simulink model "Lab_4_EBD_ibrahim"  (R2016b)
settings: Solver=VariableStepAuto  StartTime=0.0  StopTime=6  MaxStep=0.00005  RelTol=1e-3
undefined symbols (not defined in the file): F_human_max, F_rated_wheel, k, Lever_ratio, P_servo_max, R_master, R_servo, s_rated_wheel, V_initial
libraries: sdl_lib x9, nesl_utility x6, simulink x1
settings Model: Creator=AHMED MOHSEN  LastModifiedBy=AHMED MOHSEN
settings DataIOCC: ReturnWorkspaceOutputs=on
settings DebuggingCC: UnconnectedInputMsg=none  UnconnectedOutputMsg=none  UnconnectedLineMsg=none
settings ModelReferenceCC: EnableRefExpFcnMdlSchedulingChecks=off
settings SFSimCC: SimUseLocalCustomCode=on
settings RTWCC: RTWUseLocalCustomCode=on

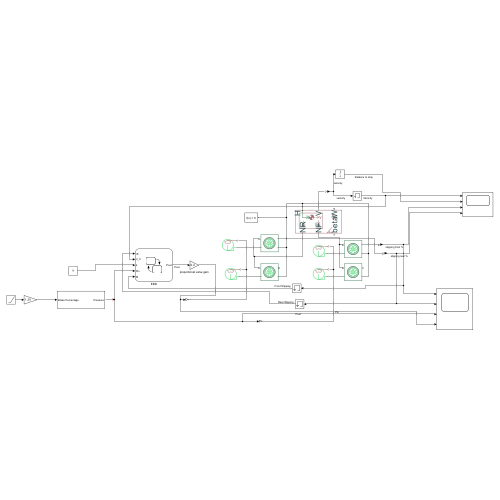
[thumbnail: Simulink's stored preview of the top-level diagram]
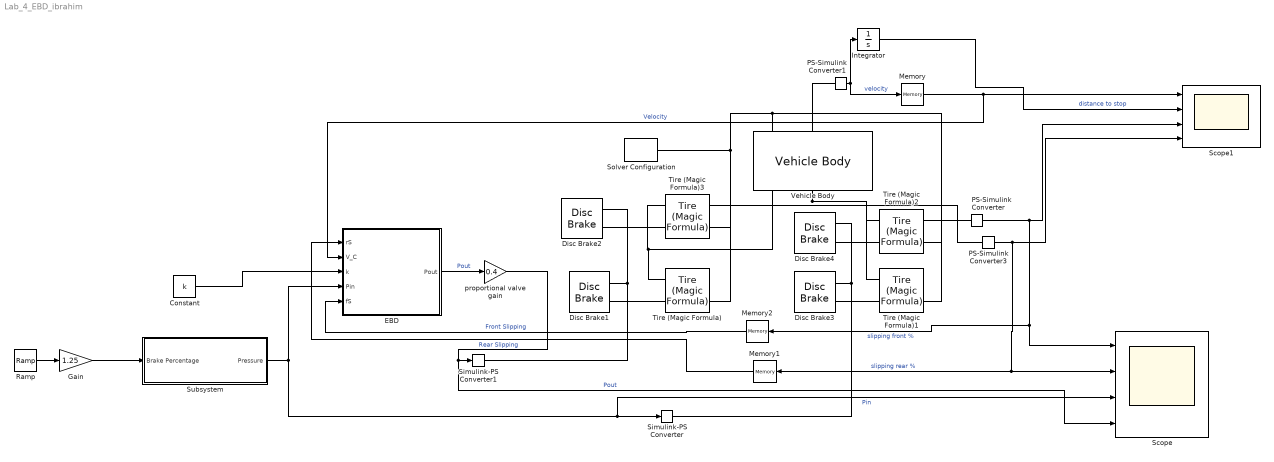
== system Lab_4_EBD_ibrahim ==
  Constant : Constant  Value=k
  Disc Brake1 : sdl_lib/Brakes & Detents/Rotational/Disc Brake  r_mean=R_disk mm  bore=D_cylinder mm  n_pads=2  thermal_port=simscape.enum.thermaleffects.omit  mu_static=0.9  mu_coulomb=0.7  temperature_TLU=[280, 300, 320] K  mu_static_TLU=[.9, .8, .7]  mu_coulomb_TLU=[.8, .7, .6]  brkwy_vel=0.1 rad/s  visc_coef=Visc_coeff N*m*s/rad  enable_faults=simscape.enum.onoff.off  faulted_pressure=0 bar  external_fault=simscape.enum.onoff.off  temporal_fault=simscape.enum.onoff.off  fault_time=5 s  report_fault=simscape.enum.assert.action.none  thermal_mass=50 kJ/K  temperature_specify=off  temperature_priority=High  temperature=300 K  temperature_nominal_specify=off  temperature_nominal_unit=K  temperature_nominal_value=1
  Disc Brake2 : sdl_lib/Brakes & Detents/Rotational/Disc Brake  r_mean=R_disk mm  bore=D_cylinder mm  n_pads=2  thermal_port=simscape.enum.thermaleffects.omit  mu_static=0.9  mu_coulomb=0.7  temperature_TLU=[280, 300, 320] K  mu_static_TLU=[.9, .8, .7]  mu_coulomb_TLU=[.8, .7, .6]  brkwy_vel=0.1 rad/s  visc_coef=Visc_coeff N*m*s/rad  enable_faults=simscape.enum.onoff.off  faulted_pressure=0 bar  external_fault=simscape.enum.onoff.off  temporal_fault=simscape.enum.onoff.off  fault_time=5 s  report_fault=simscape.enum.assert.action.none  thermal_mass=50 kJ/K  temperature_specify=off  temperature_priority=High  temperature=300 K  temperature_nominal_specify=off  temperature_nominal_unit=K  temperature_nominal_value=1
  Disc Brake3 : sdl_lib/Brakes & Detents/Rotational/Disc Brake  r_mean=R_disk mm  bore=D_cylinder mm  n_pads=2  thermal_port=simscape.enum.thermaleffects.omit  mu_static=0.9  mu_coulomb=0.7  temperature_TLU=[280, 300, 320] K  mu_static_TLU=[.9, .8, .7]  mu_coulomb_TLU=[.8, .7, .6]  brkwy_vel=0.1 rad/s  visc_coef=Visc_coeff N*m*s/rad  enable_faults=simscape.enum.onoff.off  faulted_pressure=0 bar  external_fault=simscape.enum.onoff.off  temporal_fault=simscape.enum.onoff.off  fault_time=5 s  report_fault=simscape.enum.assert.action.none  thermal_mass=50 kJ/K  temperature_specify=off  temperature_priority=High  temperature=300 K  temperature_nominal_specify=off  temperature_nominal_unit=K  temperature_nominal_value=1
  Disc Brake4 : sdl_lib/Brakes & Detents/Rotational/Disc Brake  r_mean=R_disk mm  bore=D_cylinder mm  n_pads=NO_brake_pads  thermal_port=simscape.enum.thermaleffects.omit  mu_static=0.9  mu_coulomb=0.7  temperature_TLU=[280, 300, 320] K  mu_static_TLU=[.9, .8, .7]  mu_coulomb_TLU=[.8, .7, .6]  brkwy_vel=0.1 rad/s  visc_coef=Visc_coeff N*m*s/rad  enable_faults=simscape.enum.onoff.off  faulted_pressure=0 bar  external_fault=simscape.enum.onoff.off  temporal_fault=simscape.enum.onoff.off  fault_time=5 s  report_fault=simscape.enum.assert.action.none  thermal_mass=50 kJ/K  temperature_specify=off  temperature_priority=High  temperature=300 K  temperature_nominal_specify=off  temperature_nominal_unit=K  temperature_nominal_value=1
  EBD : Stateflow chart  TreatAsAtomicUnit=on
  Gain : Gain  Gain=1.25
  Integrator : Integrator
  Memory : Memory  X0=V_initial/3.6  InheritSampleTime=on
  Memory1 : Memory  InheritSampleTime=on
  Memory2 : Memory  InheritSampleTime=on
  PS-Simulink Converter : nesl_utility/PS-Simulink Converter  PhysicalDomain=network_engine_domain  SubClassName=ps_output  LeftPortType=input  RightPortType=output  PseudoPeriodic=off  Frequencies=[]  VectorFormat=1-D array  Unit=inherit  AffineConversion=off
  PS-Simulink Converter1 : nesl_utility/PS-Simulink Converter  PhysicalDomain=network_engine_domain  SubClassName=ps_output  LeftPortType=input  RightPortType=output  PseudoPeriodic=off  Frequencies=[]  VectorFormat=inherit  Unit=m/s  AffineConversion=off
  PS-Simulink Converter3 : nesl_utility/PS-Simulink Converter  PhysicalDomain=network_engine_domain  SubClassName=ps_output  LeftPortType=input  RightPortType=output  PseudoPeriodic=off  Frequencies=[]  VectorFormat=1-D array  Unit=inherit  AffineConversion=off
  Ramp : simulink/Sources/Ramp  slope=1  start=0  X0=0
  Scope : Scope  NumInputPorts=4
  Scope1 : Scope  NumInputPorts=4
  Simulink-PS Converter : nesl_utility/Simulink-PS Converter  PhysicalDomain=network_engine_domain  SubClassName=ps_input  LeftPortType=input  RightPortType=output  PseudoPeriodic=off  Frequencies=[]  NoiseDistribution=none  NoiseParameters=[]  Unit=Pa  AffineConversion=off  FilteringAndDerivatives=provide  SimscapeFilterOrder=1  InputFilterTimeConstant=0.001  UdotUserProvided=0
  Simulink-PS Converter1 : nesl_utility/Simulink-PS Converter  PhysicalDomain=network_engine_domain  SubClassName=ps_input  LeftPortType=input  RightPortType=output  PseudoPeriodic=off  Frequencies=[]  NoiseDistribution=none  NoiseParameters=[]  Unit=Pa  AffineConversion=off  FilteringAndDerivatives=provide  SimscapeFilterOrder=1  InputFilterTimeConstant=0.001  UdotUserProvided=0
  Solver Configuration : nesl_utility/Solver Configuration  PhysicalDomain=network_engine_domain  SubClassName=solver  LeftPortType=input  RightPortType=generic  Tones=[]  Harmonics=[]  SimulateNoise=off  Profile=off  UseLocalSampling=off  EnableSwitchedLinearOptims=on  FrequencyDomain=off  UseCCode=off  RelTol=0.001  AbsTol=0.001  MinStep=1e-09  ToWorkspace=off  RevertToSquareIcSolve=off  NumHomotopyIterations=100  PhasorMode=off  PhasorModeNumHarmonics=1  ConsistencySolver=NEWTON_XTOL_AFTER_FTOL  IndexReductionMethod=DerivativeReplacement  DoDC=off  ResidualTolerance=1e-09  ConsistencyTolSource=GLOBAL  ConsistencyAbsTol=0.001  ConsistencyRelTol=0.001  ConsistencyTolFactor=0.001  UseLocalSolver=off  LocalSolverChoice=NE_BACKWARD_EULER_ADVANCER  ResolveIndetEquations=on  FunctionEvalNumThread=1  LocalSolverSampleTime=0.001  DoFixedCost=off  MaxNonlinIter=3  MaxModeIter=2  ComputeImpulses=off  ImpulseIterations=2  LinearAlgebra=auto  LinearAlgebraNumThread=0  EquationFormulation=NE_TIME_EF  DelaysMemoryBudget=1024  AutomaticFiltering=on  FilteringTimeConstant=0.001  PartitionStorageMethod=AS_NEEDED  PartitionMemoryBudget=1024  PartitionMethod=ROBUST  MultibodyUseLocalSolver=off  MultibodyLocalSolverChoice=ODE1  MultibodyLocalSolverSampleTime=0.001
  Subsystem : Subsystem
  Tire (Magic Formula){,1..3} (4 alike) : sdl_lib/Tires & Vehicles/Tire (Magic Formula)  parameterization=sdl.enum.magic_tire_model.peak  F_z1=F_rated_wheel N  F_x1=F_rated_wheel*s_rated_wheel N  kappa1=10  B_m=10  C_m=1.9  D_m=1  E_m=0.97  fz0=4000 N  p_Cx=1.685  p_Dx=[1.21, -.037]  p_Ex=[.344, .095, -.02, 0]  p_Kx=[21.51, -.163, .245]  p_Hx=[-.002, .002]  p_Vx=[0, 0]  rolling_radius_model=sdl.enum.RollingRadiusParameterization.Constant  r_e=R_wheel m  r_0=0.3 m  breff=8.39  dreff=0.26  freff=0.074  q_re0=0.99  q_v1=0.008  longvl=17 m/s  cz=5e5 N/m  model_resistance=false  resistance_model=sdl.enum.rollingResistanceParameterization.constant  coeff=0.015  p_tire=250e3 Pa  alpha=-0.003  beta=0.97  coeff_a=84e-4  coeff_b=6.2e-4 s/m  coeff_c=1.6e-4 s^2/m^2  p_tire0=240e3 Pa  fz0_resistance=4000 N  vH0=16 m/s  q_Sy=[.0082, 0, .0014, .001, 0, 0, 1.08, -.5]  v_thr=0.001 m/s  enable_scaling_coefficients=false  lfzO=1  lcx=1  lmux=1  lex=1  lkx=1  lhx=1  lvx=1  lmy=1  model_compliance=sdl.enum.compliance.off  stiffness=1e6 N/m  damping=1000 N*s/m  model_inertia=sdl.enum.model_inertia.on  inertia=1 kg*m^2  initial_velocity=V_initial/3.6/R_wheel rad/s  vxlow=1 m/s  v_tr_thr=0.1 m/s  kpumin=-1.5  kpumax=1.5
  Vehicle Body : sdl_lib/Tires & Vehicles/Vehicle Body  mass=m_vehicle kg  n_w=2  x_f=f_CG m  x_r=r_CG m  y_c=h_CG m  mass_var=simscape.enum.onoff.off  g=9.81 m/s^2  liftoff_warning=simscape.enum.onoff.off  area=3 m^2  Cd=Drag_coeff  rho=1.18 kg/m^3  model_pitch=simscape.enum.onoff.off  inertia=4000 kg*m^2  suspension_model=sdl.enum.linearTLU.linear  k_f=1e4 N/m  b_f=1e4 N*s/m  k_r=1e4 N/m  b_r=1e4 N*s/m  k_f_TLU=[-2000, -1000, 0, 1000, 2000] N  x_f_TLU=[-.4, -.2, 0, .2, .4] m  b_f_TLU=[-200, -100, 0, 100, 200] N  v_f_TLU=[-4, -2, 0, 2, 4] m/s  k_r_TLU=[-2000, -1000, 0, 1000, 2000] N  x_r_TLU=[-.4, -.2, 0, .2, .4] m  b_r_TLU=[-200, -100, 0, 100, 200] N  v_r_TLU=[-4, -2, 0, 2, 4] m/s  interp_method=simscape.enum.interpolation.linear  extrap_method=simscape.enum.extrapolation.linear  model_hardstop=simscape.enum.onoff.off  upper_bound_f=.25 m  lower_bound_f=-.25 m  stop_k_f=1e6 N/m  stop_b_f=150 N*s/m  upper_bound_r=.25 m  lower_bound_r=-.25 m  stop_k_r=1e6 N/m  stop_b_r=150 N*s/m  initial_pitch=0 rad  initial_pitch_rate=0 rad/s  v_specify=on  v_priority=High  v=V_initial kph  v_nominal_specify=off  v_nominal_unit=m/s  v_nominal_value=1
  proportional valve gain : Gain  Gain=0.4
  wires:
  EBD/1(Pout) -> proportional valve gain/1  "Pout"
  Memory/1 -> EBD/2(V_C), Scope1/1  "Velocity"
  Memory2/1 -> EBD/5(fS)  "Front Slipping"
  PS-Simulink Converter3/1 -> Scope1/4, Scope/2, Memory1/1  "slipping rear %"
  Ramp/1 -> Gain/1
  proportional valve gain/1 -> Scope/4, Simulink-PS Converter1/1  "Pout"
  Constant/1 -> EBD/3(k)
  PS-Simulink Converter/1 -> Memory2/1, Scope/1, Scope1/3  "slipping front %"
  Integrator/1 -> Scope1/2  "distance to stop"
  PS-Simulink Converter1/1 -> Memory/1, Integrator/1  "velocity"
  Subsystem/1(Pressure) -> EBD/4(Pin), Scope/3, Simulink-PS Converter/1  "Pin"
  Memory1/1 -> EBD/1(rS)  "Rear Slipping"
  Gain/1 -> Subsystem/1(Brake Percentage)
  connections:
  Disc Brake4/LConn1 -- Disc Brake3/LConn1 -- Simulink-PS Converter/RConn1
  Solver Configuration/RConn1 -- Tire (Magic Formula)/RConn2 -- Tire (Magic Formula)3/RConn2 -- Vehicle Body/LConn1 -- Tire (Magic Formula)1/RConn2 -- Tire (Magic Formula)2/RConn2
  Tire (Magic Formula)/LConn1 -- Vehicle Body/RConn1 -- Tire (Magic Formula)3/LConn1
  Disc Brake2/LConn1 -- Disc Brake1/LConn1 -- Simulink-PS Converter1/RConn1
  Vehicle Body/RConn2 -- Tire (Magic Formula)1/LConn1 -- Tire (Magic Formula)2/LConn1
  Disc Brake1/LConn2 -- Tire (Magic Formula)/LConn2
  Tire (Magic Formula)3/RConn1 -- PS-Simulink Converter3/LConn1
  Vehicle Body/LConn2 -- PS-Simulink Converter1/LConn1
  Disc Brake3/LConn2 -- Tire (Magic Formula)1/LConn2
  PS-Simulink Converter/LConn1 -- Tire (Magic Formula)2/RConn1
  Disc Brake4/LConn2 -- Tire (Magic Formula)2/LConn2
  Disc Brake2/LConn2 -- Tire (Magic Formula)3/LConn2

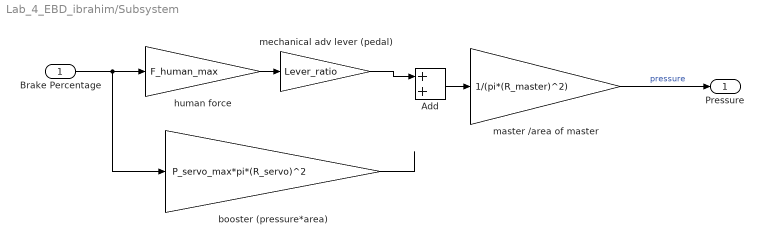
== system Lab_4_EBD_ibrahim/Subsystem ==
  Brake Percentage : Inport
  Add : Sum
  booster (pressure*area) : Gain  Gain=P_servo_max*pi*(R_servo)^2
  human force : Gain  Gain=F_human_max
  master /area of master : Gain  Gain=1/(pi*(R_master)^2)
  mechanical adv lever (pedal) : Gain  Gain=Lever_ratio
  Pressure : Outport
  wires:
  human force/1 -> mechanical adv lever (pedal)/1
  Brake Percentage/1 -> human force/1, booster (pressure*area)/1
  mechanical adv lever (pedal)/1 -> Add/1
  Add/1 -> master /area of master/1
  master /area of master/1 -> Pressure/1  "pressure"
  booster (pressure*area)/1 -> ?

== stateflow chart Lab_4_EBD_ibrahim/EBD ==
  state active
    state hold
      during:
      Pout=Pout;
    state increase
      during:
      Pout=Pout*k;
    (default) -> increase
    increase -> hold : [rS<fS | rS-fS==0.01]
    hold -> increase : [rS>fS]
  state passive
    entry:
    Pout=Pin
    during:
    Pout=Pin;
  passive -> active : [rS<-0.02]
  (default) -> passive
  active -> passive : [V_C<0.0001]
  data: rS input; V_C input; k input; Pin input; Pout output; fS input
